simulink model "Control_Lab"  (R2021b)
settings: Solver=daessc  StartTime=0.0  StopTime=10  RelTol=1e-3  AbsTol=1e-3  EnableMultiTasking=on
model workspace (MAT data in the model file):
  iz = [0.192  0.091; 0.207  0.094; 0.221  0.104; 0.238  0.118; 0.251  0.141; 0.262  0.168; 0.268  0.205; 0.27  0.242; 0.267  0.277; 0.262  0.308; 0.246  0.348; 0.232  0.369; 0.206  0.39; 0.185  0.39; 0.16  0.377; 0.137  0.349; 0.126  0.325; 0.118  0.297; 0.114  0.265; 0.113  0.237; 0.118  0.191; 0.128  0.156; 0.139  0.13; 0.156  0.107; 0.175  0.096]
  one = [0.064  0.072; 0.088  0.03; 0.169  0.03; 0.168  0.458; 0.129  0.458; 0.128  0.073]
  smiData.RigidTransform.translation = [-21.5561986301 -14.8674859839 15.0728144895]
  smiData.RigidTransform.angle = 0
  smiData.RigidTransform.axis = [0 0 0]
  smiData.RigidTransform.ID = 'RootGround[rack-1]'
  smiData.Solid.mass = 0.0200061588425
  smiData.Solid.CoM = [0 0.838779102261 -0.00603396973069]
  smiData.Solid.MoI = [0.670200057653 0.669872690066 0.00366172739385]
  smiData.Solid.PoI = [5.56695055283e-05 0 0]
  smiData.Solid.color = [0.792156862745 0.819607843137 0.933333333333]
  smiData.Solid.opacity = 1
  smiData.Solid.ID = 'rack*:*Default'
  three = [0.252  0.12; 0.239  0.091; 0.214  0.068; 0.179  0.053; 0.14  0.052; 0.107  0.064; 0.083  0.082; 0.065  0.121; 0.075  0.155; 0.102  0.176; 0.129  0.188; 0.163  0.194; 0.182  0.194; 0.183  0.24; 0.131  0.247; 0.099  0.256; 0.068  0.28; 0.048  0.313; 0.047  0.345; 0.055  0.378; 0.084  0.41; 0.127  0.429; 0.179  0.43; 0.214  0.419; 0.246  0.396; 0.26  0.368; 0.269  0.344; 0.311  0.344; 0.303  0.374; 0.29  0.409; 0.262  0.442; 0.23  0.463; 0.18  0.475; 0.137  0.476; 0.097  0.465; 0.057  0.441; 0.028  0.411; 0.011  0.374; 0.006  0.353; 0.01  0.295; 0.028  0.258; 0.05  0.233; 0.08  0.214; 0.06  0.196; 0.041  0.175; 0.029  0.135; 0.029  0.104; 0.043  0.066; 0.074  0.032; 0.106  0.015; 0.147  0.006; 0.187  0.007; 0.223  0.021; 0.255  0.044; 0.278  0.081; 0.294  0.119]
  two = [0.081  0.154; 0.042  0.154; 0.05  0.108; 0.06  0.085; 0.082  0.055; 0.106  0.033; 0.135  0.02; 0.161  0.013; 0.194  0.014; 0.226  0.02; 0.253  0.032; 0.279  0.054; 0.297  0.083; 0.305  0.109; 0.309  0.141; 0.306  0.168; 0.299  0.189; 0.281  0.221; 0.242  0.271; 0.119  0.401; 0.315  0.403; 0.314  0.445; 0.027  0.446; 0.242  0.214; 0.263  0.177; 0.272  0.145; 0.264  0.106; 0.243  0.079; 0.208  0.059; 0.185  0.058; 0.162  0.06; 0.133  0.067; 0.12  0.076; 0.102  0.092; 0.088  0.119; 0.085  0.134]
  xy_simple = [39.1661  19.7032018238; 3.8339  19.7032; -0.28263658  19.7032; -0.28263658  0; 43  0; 43  19.7032]
  zero = [0.2  0.026; 0.245  0.033; 0.288  0.063; 0.316  0.099; 0.335  0.149; 0.345  0.197; 0.347  0.246; 0.344  0.292; 0.338  0.339; 0.324  0.384; 0.3  0.429; 0.269  0.456; 0.223  0.475; 0.173  0.475; 0.132  0.46; 0.097  0.426; 0.072  0.383; 0.062  0.338; 0.058  0.289; 0.058  0.242; 0.059  0.192; 0.068  0.145; 0.083  0.102; 0.111  0.062; 0.149  0.037]
undefined symbols (not defined in the file): X, Y, Z
libraries: sm_lib x1357, nesl_utility x28, slpidlib x5
(part 1 of 28)
settings Model: Creator=acontr14  LastModifiedBy=acontr14
settings SolverCC: AutoScaleAbsTol=off  AlgebraicLoopSolver=TrustRegion
settings DataIOCC: LimitDataPoints=on  MaxDataPoints=10000
settings OptimizationCC: LifeSpan=inf
settings DebuggingCC: AllowSymbolicDim=off  SFUnexpectedBacktrackingDiag=warning  SFNoUnconditionalDefaultTransitionDiag=warning  SFExecutionAtInitializationDiag=none  SFMachineParentedDataDiag=warning  ArithmeticOperatorsInVariantConditions=warning
settings SFSimCC: SimUseLocalCustomCode=off  CustomCodeUndefinedFunction=UseInterfaceOnly
settings RTWCC: RTWUseLocalCustomCode=off
settings CodeAppCC: StateflowObjectComments=on
settings GRTTargetCC: TargetLangStandard=C89/C90 (ANSI)
settings ConfigComp: CovMetricSettings=dw  CovSaveCumulativeToWorkspaceVar=on  CovSaveSingleToWorkspaceVar=on  CovExternalEMLEnable=off  CovSFcnEnable=off
settings SimscapeCC: SimscapeLogType=all  SimscapeLogSimulationStatistics=on  SimscapeLogDataHistory=10000

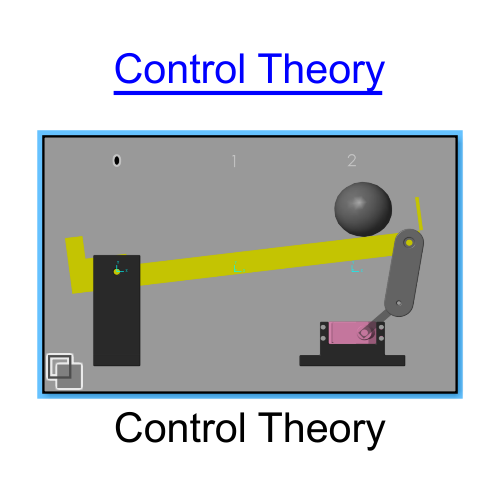
[thumbnail: Simulink's stored preview of the top-level diagram]
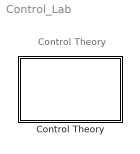
== system Control_Lab ==
  note: Control Theory
  Control Theory : Subsystem  Variant=on  VariantControlMode=label  VariantControl=ConTh  LabelModeActiveChoice=PIDBC
      mask Display: image('$imagefile'); % Use "Edit Image" on toolstrip to change.

== system Control_Lab/Control Theory ==
  note: PID Controlled Disc
  note: 1 Mass 1 Spring
  note: PID Ball Control
  note: PID Pendulum
  note: Cart Disturbance
  1 DOF PID : Subsystem  VariantControl=dof1PID  mask{materials=PLA, GG=3.5, b_den1=1.25, d_den=1.25, d=.000002, ll=114.0, load=off, lmass=5, dmass=27.0, pos1=50, zerodis=on, zero_forces=off, force_type=Harmonic, Force=5, Har_Force=2, freq=5, Pulse_Force=2, Pulse_Period=3, Pulse_Width=5, PID_source=Square, sin_amp=30, sin_freq=1, squ_amp=50, squ_freq=.2, step_mag=30}
      mask prompts: materials "Choose Material of Rod:"; GG "Shear Modulus (GPa):"; b_den1 "Density of Rod (g/cm^3):"; d_den "Density of Disc (g/cm^3):"; d "Rod Damping"; ll "Position of Disc (mm):"; load "Add Load"; lmass "Load Mass (kg)"; dmass "Distance from Center (mm)"; pos1 "Initial Rotation of Disc (deg):"; zerodis "Zero Initial Displacement"; zero_forces "Zero Forces"; force_type "Force Response Type"; Force "Magnitude (N):"; Har_Force "Magnitude (N):"; freq "Frequency (rad/s):"; Pulse_Force "Magnitude (N):"; Pulse_Period "Period (sec):"; Pulse_Width "Pulse Width (% of period):"; PID_source "Angle Signal"; sin_amp "Amplitude (deg):"; sin_freq "Frequency (rad/sec):"; squ_amp "Amplitude (deg):"; squ_freq "Frequency (Hz):"; step_mag "Magnitude (deg):"
      mask init:
      | switch materials
      |     case 1
      |         G= 1; %GPa
      |         b_den= 1; %g/cm^3
      |     case 2
      |         G= 3.5;
      |         b_den= 1.24;
      |     case 3
      |         G= GG;
      |         b_den= b_den1;
      | end
      | switch force_type
      |     case 1
      |         Har_Force = 0;
      |         freq = 0;
      |         Pulse_Force = 0;
      |     case 2
      |         Force = 0;
      |         Pulse_Force = 0;
      |     case 3
      |         Har_Force = 0;
      |         freq = 0;
      |         Force = 0;
      | end
      | if zero_forces == 1
      |     Har_Force = 0;
      |     Force = 0;
      |     freq = 0;
      | end
      | if zerodis == 1
      |     pos1 = 0;
      | end
      | switch PID_source
      |     case 1
      |         set_param('Control_Lab/Control Theory/1 DOF PID/Sine Wave2','Commented','off');
      |         set_param('Control_Lab/Control Theory/1 DOF PID/Signal Generator','Commented','on');
      |         set_param('Control_Lab/Control Theory/1 DOF PID/Step2','Commented','on');
      |     case 2
      |         set_param('Control_Lab/Control Theory/1 DOF PID/Sine Wave2','Commented','on');
      |         set_param('Control_Lab/Control Theory/1 DOF PID/Signal Generator','Commented','off');
      |         set_param('Control_Lab/Control Theory/1 DOF PID/Step2','Commented','on');
      |     case 3
      |         set_param('Control_Lab/Control Theory/1 DOF PID/Sine Wave2','Commented','on');
      |         set_param('Control_Lab/Control Theory/1 DOF PID/Signal Generator','Commented','on');
      |         set_param('Control_Lab/Control Theory/1 DOF PID/Step2','Commented','off');
      | end
      | % l1=65e-3; l2=l1; l3=l1; l4=l1;
      | l=ll*10^-3;
      | l2=.2025-l;
      | G=G*10^9;
      | dd=2.25e-3;
      | k1=pi*G*dd^4/(32*l);
      | k2=(pi*G*dd^4/(32*l2));
      | % k3=(pi*G*dd^4/(32*l3));
      | kt1=k1+k2;
      | % kt2=k2+k3;
      | % kt3=2*k3;
      mask TypeOptions materials: Steel | PLA | Enter Material Properties
      mask Callback materials:
      | % Get the mask parameter values. This is a cell
      | %   array of character vectors.
      | maskStr = get_param(gcb,'materials');
      | 
      | % The pop-up menu is the first mask parameter.
      | %   Check the value selected in the pop-up
      | if strcmp(maskStr(1),'E'),
      | 
      |     % Set the visibility of both parameters on when
      |     %   User-defined is selected in the pop-up.
      | 
      |     set_param(gcb,'MaskVisibilities',{'on';'on';'on';'on';'on';'on';'on';'on';'on';'on';'on';'on';'on';'on';'on';'on';'on';'on';'on';'on';'on';'on';'on';'on';'on'}),
      | 
      | else
      | 
      |     % Turn off the visibility of the Value field
      |     %   when User-defined is not selected.
      | 
      |     set_param(gcb,'MaskVisibilities',{'on';'off';'off';'on';'on';'on';'on';'on';'on';'on';'on';'on';'on';'on';'on';'on';'on';'on';'on';'on';'on';'on';'on';'on';'on'}),
      | 
      |     % Set the character vector in the Values field equal to the
      |     % character vector selected in the Gain pop-up menu.
      | end
      mask Callback load:
      | load = get_param(gcb,'load');
      | if strcmp(load,'on')
      |     set_param('Control_Lab/Control Theory/1 DOF PID/Cylindrical Solid','Commented','off');
      |     set_param('Control_Lab/Control Theory/1 DOF PID/Rigid Transform9','Commented','off');
      |     set_param('Control_Lab/Control Theory/1 DOF PID/Cylindrical Solid1','Commented','off');
      |     set_param('Control_Lab/Control Theory/1 DOF PID/Rigid Transform7','Commented','off');
      | else
      |     set_param('Control_Lab/Control Theory/1 DOF PID/Cylindrical Solid','Commented','on');
      |     set_param('Control_Lab/Control Theory/1 DOF PID/Rigid Transform9','Commented','on');
      |     set_param('Control_Lab/Control Theory/1 DOF PID/Cylindrical Solid1','Commented','on');
      |     set_param('Control_Lab/Control Theory/1 DOF PID/Rigid Transform7','Commented','on');
      | end
      mask Callback zero_forces:
      | % Enable and disable parameters
      | 
      | % Get the value of the Enable Bias checkbox
      | % unchecked = 'off'
      | % checked = 'on'
      | enab = get_param(gcb,'zero_forces');
      | 
      | % Set the 'MaskEnables' property for each parameters
      | if strcmp(enab,'on')
      |     set_param(gcb,'MaskEnables',{'on','on','on','on','on','on','on','on','on','on','on','on','off','off','off','off','off','off','off','on','on','on','on','on','on'});
      | else
      |     set_param(gcb,'MaskEnables',{'on','on','on','on','on','on','on','on','on','on','on','on','on','on','on','on','on','on','on','on','on','on','on','on','on'});
      | end
      | 
      | % Note that the value of the bias is not handled here.
      | % See the Initialization tab
      mask TypeOptions force_type: Step | Harmonic | Pulse
      mask TypeOptions PID_source: Harmonic | Square | Constant
      mask DialogControl Control4 Prompt: Update Model
      mask DialogControl Control4 Callback: set_param(bdroot,'SimulationCommand','update')
      mask DialogControl Control3 Prompt: Run Simulation
      mask DialogControl Control3 Callback: set_param(bdroot,'SimulationCommand','start')
      mask DialogControl Control5 Prompt: Stop Simulation
      mask DialogControl Control5 Callback: set_param(bdroot,'SimulationCommand','stop')
      mask DialogControl Control2 Prompt: Open Position Plot
      mask DialogControl Control2 Callback: open(Simulink.BlockPath({'Control_Lab/Control Theory/1 DOF PID/Scope1'}))
      mask DialogControl Control7 Prompt: Open PID Controller
      mask DialogControl Control7 Callback: open(Simulink.BlockPath({'Control_Lab/Control Theory/1 DOF PID/PID Controller'}))
      mask DialogControl Container8 Prompt: Parameters
      mask DialogControl Container14 Prompt: Loading
      mask DialogControl Container13 Prompt: Free Response
      mask DialogControl Container17 Prompt: Force Response
      mask DialogControl Container18 Prompt: Step Response
      mask DialogControl Container19 Prompt: Harmonic Response
      mask DialogControl Container23 Prompt: Pulse
      mask DialogControl Container16 Prompt: PID Desired Angle
      mask DialogControl Container20 Prompt: Harmonic
      mask DialogControl Container21 Prompt: Square
      mask DialogControl Container22 Prompt: Constant
      mask Display: image('$imagefile'); % Use "Edit Image" on toolstrip to change.
  Cart Disturbance : Subsystem  VariantControl=CartDist  mask{rodlength=10, m=10}
      mask prompts: rodlength "Rod Length (cm)"; m "Pendulum Mass (kg)"
      mask DialogControl Control4 Prompt: Update Model
      mask DialogControl Control4 Callback: set_param(bdroot,'SimulationCommand','update')
      mask DialogControl Control5 Prompt: Run Simulation
      mask DialogControl Control5 Callback: set_param(bdroot,'SimulationCommand','start')
      mask DialogControl Control6 Prompt: STOP Simulation
      mask DialogControl Control6 Callback: set_param(bdroot,'SimulationCommand','stop')
      mask DialogControl Control2 Prompt: PID Control
      mask DialogControl Control2 Callback: open(Simulink.BlockPath({'Control_Lab/Control Theory/Cart Disturbance/PID Controller'}))
      mask DialogControl Control3 Prompt: Position Scope
      mask DialogControl Control3 Callback: open(Simulink.BlockPath({'Control_Lab/Control Theory/Cart Disturbance/Scope1'}))
  Mass Spring1 : Subsystem  AncestorBlock=Lib/Mass Spring  VariantControl=11ms  mask{m1=2, k1=600, d1=1, s_f=.35, id1=-0.350, zero_forces=off, zerodis=on, force_type=Harmonic, Force=4, Har_Force=5, freq=(2*pi)*1, PID_source=Square, sin_amp=0.560, sin_freq=(2*pi)/1, squ_amp=2, squ_freq=.5, step_mag=2}
      mask prompts: m1 "Mass1 (kg)"; k1 "K1 Spring Constant (N/m)"; d1 "Spring Damping (kg/s)"; s_f "Surface Friction (N/(m/s))"; id1 "M1 Initial Displacement (cm)"; zero_forces "Zero Forces"; zerodis "Zero Initial Displacement"; force_type "Force Response Type"; Force "Magnitude(N)"; Har_Force "Magnitude(N)"; freq "Frequency(rad/s)"; PID_source "Position Signal"; sin_amp "Amplitude (cm):"; sin_freq "Frequency (rad/sec):"; squ_amp "Amplitude (cm):"; squ_freq "Frequency (Hz):"; step_mag "Magnitude (cm):"
      mask init:
      | switch force_type
      |     case 1
      |         Har_Force = 0;
      |         freq = 0;
      |     case 2
      |         Force = 0;
      | end
      | if zero_forces == 1
      |     Har_Force = 0;
      |     Force = 0;
      |     freq = 0;
      | end
      | 
      | if zerodis == 1
      |     id1 = 0;
      | end
      | switch PID_source
      |     case 1
      |         set_param('Control_Lab/Control Theory/Mass Spring1/Sine Wave3','Commented','off');
      |         set_param('Control_Lab/Control Theory/Mass Spring1/Signal Generator','Commented','on');
      |         set_param('Control_Lab/Control Theory/Mass Spring1/Step2','Commented','on');
      |     case 2
      |         set_param('Control_Lab/Control Theory/Mass Spring1/Sine Wave3','Commented','on');
      |         set_param('Control_Lab/Control Theory/Mass Spring1/Signal Generator','Commented','off');
      |         set_param('Control_Lab/Control Theory/Mass Spring1/Step2','Commented','on');
      |     case 3
      |         set_param('Control_Lab/Control Theory/Mass Spring1/Sine Wave3','Commented','on');
      |         set_param('Control_Lab/Control Theory/Mass Spring1/Signal Generator','Commented','on');
      |         set_param('Control_Lab/Control Theory/Mass Spring1/Step2','Commented','off');
      | end
      mask Callback zero_forces:
      | % Enable and disable parameters
      | 
      | % Get the value of the Enable Bias checkbox
      | % unchecked = 'off'
      | % checked = 'on'
      | enab = get_param(gcb,'zero_forces');
      | 
      | % Set the 'MaskEnables' property for each parameters
      | if strcmp(enab,'on')
      |     set_param(gcb,'MaskVisibilities',{'on','on','on','on','on','on','off','off','off','off','off','on','on','on','on','on','on'});
      | else
      |     set_param(gcb,'MaskVisibilities',{'on','on','on','on','on','on','on','on','on','on','on','on','on','on','on','on','on'});
      | end
      | 
      | % Note that the value of the bias is not handled here.
      | % See the Initialization tab
      mask Callback zerodis:
      | % Enable and disable parameters
      | 
      | % Get the value of the Enable Bias checkbox
      | % unchecked = 'off'
      | % checked = 'on'
      | enab = get_param(gcb,'zerodis');
      | 
      | % Set the 'MaskEnables' property for each parameters
      | if strcmp(enab,'on')
      |     set_param(gcb,'MaskEnables',{'on','on','on','on','off','on','on','on','on','on','on','on','on','on','on','on','on'});
      | else
      |     set_param(gcb,'MaskEnables',{'on','on','on','on','on','on','on','on','on','on','on','on','on','on','on','on','on'});
      | end
      | 
      | % Note that the value of the bias is not handled here.
      | % See the Initialization tab
      mask TypeOptions force_type: Step | Harmonic
      mask TypeOptions PID_source: Harmonic | Square | Constant
      mask DialogControl Control4 Prompt: Update Model
      mask DialogControl Control4 Callback: set_param(bdroot,'SimulationCommand','update')
      mask DialogControl Control2 Prompt: Run Simulation
      mask DialogControl Control2 Callback: set_param(bdroot,'SimulationCommand','start')
      mask DialogControl Control3 Prompt: STOP Simulation
      mask DialogControl Control3 Callback: set_param(bdroot,'SimulationCommand','stop')
      mask DialogControl Control7 Prompt: Open Scope Plot
      mask DialogControl Control7 Callback: open(Simulink.BlockPath({'Control_Lab/Control Theory/Mass Spring1/Position'}))
      mask DialogControl Control13 Prompt: Open PID Controller
      mask DialogControl Control13 Callback: open(Simulink.BlockPath({'Control_Lab/Control Theory/Mass Spring1/PID Controller'}))
      mask DialogControl Container6 Prompt: Variables
      mask DialogControl Container8 Prompt: Free Response
      mask DialogControl Container11 Prompt: Free Response
      mask DialogControl Control10 Prompt: "Check Box below for Only Free Response"
      mask DialogControl Container19 Prompt: Forced Response
      mask DialogControl Container10 Prompt: Forced Response
      mask DialogControl Control9 Prompt: Uncheck "Zero Forces" in Free Response Tab to add Forced Response
      mask DialogControl Container13 Prompt: Step Response
      mask DialogControl Container16 Prompt: Harmonic Response
      mask DialogControl Container15 Prompt: PID Desired Position
      mask DialogControl Container17 Prompt: Harmonic
      mask DialogControl Container18 Prompt: Square
      mask DialogControl Container20 Prompt: Constant
      mask Display: image('$imagefile'); % Use "Edit Image" on toolstrip to change.
  PID Ball Control : Subsystem  VariantControl=PIDBC  mask{despos=125.0}
      mask prompts: despos "Target Position (mm):"
      mask DialogControl Control5 Prompt: Update Model
      mask DialogControl Control5 Callback: set_param(bdroot,'SimulationCommand','update')
      mask DialogControl Control4 Prompt: Run Simulation
      mask DialogControl Control4 Callback: set_param(bdroot,'SimulationCommand','start')
      mask DialogControl Control3 Prompt: STOP Simulation
      mask DialogControl Control3 Callback: set_param(bdroot,'SimulationCommand','stop')
      mask DialogControl Control2 Prompt: Open Scope Plot
      mask DialogControl Control2 Callback: open(Simulink.BlockPath({'Control_Lab/Control Theory/PID Ball Control/Scope'}))
      mask DialogControl Control7 Prompt: Open PID Controller
      mask DialogControl Control7 Callback: open(Simulink.BlockPath({'Control_Lab/Control Theory/PID Ball Control/PID Controller1'}))
      mask Display: image('$imagefile'); % Use "Edit Image" on toolstrip to change.
  PID Pendulum : Subsystem  VariantControl=PIDpen  mask{rodlength=.5, m1=.5, amplitude=10, pulsenumber=5, PID_source=Constant, sin_amp=30, sin_freq=(2*pi)/2, squ_amp=0, squ_freq=0, step_mag=30}
      mask prompts: rodlength "Rod Length (m):"; m1 "Mass (kg):"; amplitude "Disturbance (N):"; pulsenumber "Number of Pulses:"; PID_source "Angle Signal"; sin_amp "Amplitude (deg):"; sin_freq "Frequency (rad/sec):"; squ_amp "Amplitude (deg):"; squ_freq "Frequency (Hz):"; step_mag "Magnitude (deg):"
      mask init:
      | set_param(bdroot,'StopTime','10')
      | switch PID_source
      |     case 1
      |         set_param('Control_Lab/Control Theory/PID Pendulum/Sine Wave3','Commented','off');
      |         set_param('Control_Lab/Control Theory/PID Pendulum/Signal Generator','Commented','on');
      |         set_param('Control_Lab/Control Theory/PID Pendulum/Step2','Commented','on');
      |     case 2
      |         set_param('Control_Lab/Control Theory/PID Pendulum/Sine Wave3','Commented','on');
      |         set_param('Control_Lab/Control Theory/PID Pendulum/Signal Generator','Commented','off');
      |         set_param('Control_Lab/Control Theory/PID Pendulum/Step2','Commented','on');
      |     case 3
      |         set_param('Control_Lab/Control Theory/PID Pendulum/Sine Wave3','Commented','on');
      |         set_param('Control_Lab/Control Theory/PID Pendulum/Signal Generator','Commented','on');
      |         set_param('Control_Lab/Control Theory/PID Pendulum/Step2','Commented','off');
      | end
      mask TypeOptions PID_source: Harmonic | Square | Constant
      mask DialogControl DescGroupVar Prompt: PID Pendulum
      mask DialogControl Control4 Prompt: Update Model
      mask DialogControl Control4 Callback: set_param(bdroot,'SimulationCommand','update')
      mask DialogControl Control5 Prompt: Run Simulation
      mask DialogControl Control5 Callback: set_param(bdroot,'SimulationCommand','start')
      mask DialogControl Control6 Prompt: STOP Simulation
      mask DialogControl Control6 Callback: set_param(bdroot,'SimulationCommand','stop')
      mask DialogControl Container3 Prompt: PID Desired Angle
      mask DialogControl Container4 Prompt: Harmonic
      mask DialogControl Container6 Prompt: Square
      mask DialogControl Container5 Prompt: Constant
      mask DialogControl Control2 Prompt: PID Controller
      mask DialogControl Control2 Callback: open(Simulink.BlockPath({'Control_Lab/Control Theory/PID Pendulum/PID Controller'}))
      mask DialogControl Control3 Prompt: Angle Plot
      mask DialogControl Control3 Callback: open(Simulink.BlockPath({'Control_Lab/Control Theory/PID Pendulum/Scope1'}))
      mask Display: image('$imagefile'); % Use "Edit Image" on toolstrip to change.
